simulink model "bicycle_20230612_Plots"  (R2022b)
settings: Solver=ode1  StartTime=0.0  StopTime=60  FixedStep=1e-4  RelTol=1e-3
model workspace (MAT data in the model file):
  Mu = [0.1; 0.1; 0; 0]
  x_init = [5; 0; 0]
libraries: simulink_extras x1
settings Model: Creator=giuli  LastModifiedBy=simob

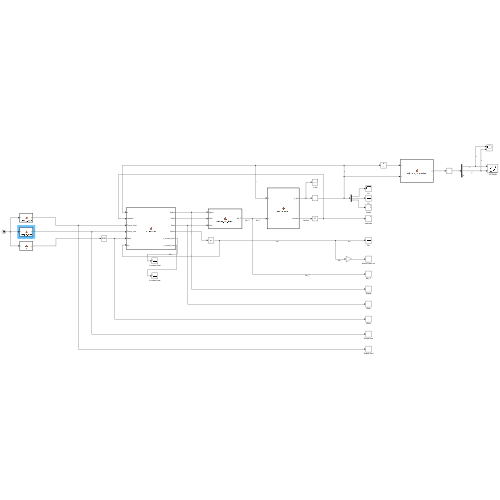
[thumbnail: Simulink's stored preview of the top-level diagram]
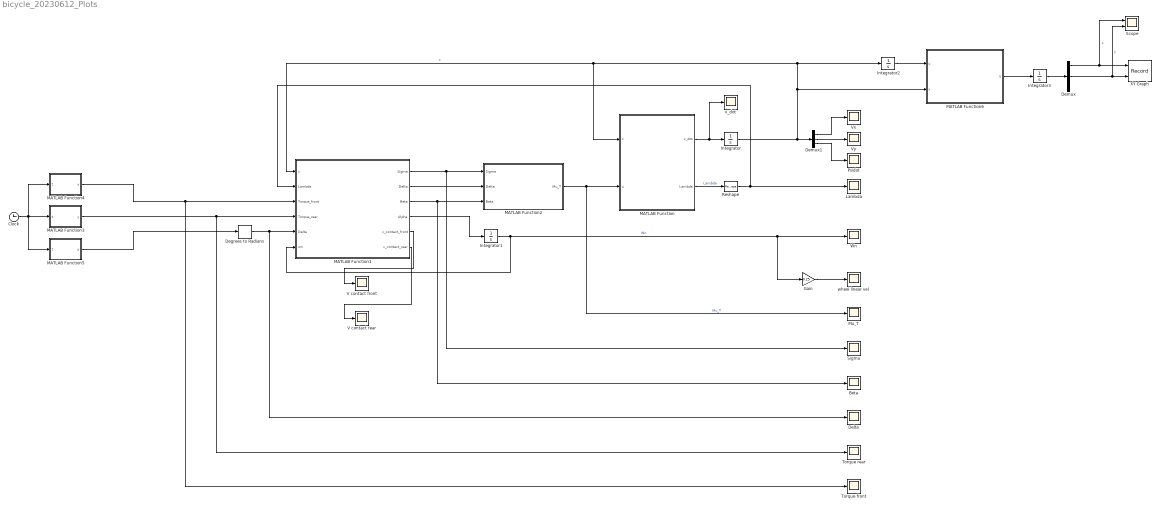
== system bicycle_20230612_Plots ==
  Beta : Scope
  Clock : Clock
  Degrees to Radians : simulink_extras/Transformations/Degrees to Radians
  Delta : Scope
  Demux : Demux  Outputs=3
  Demux1 : Demux  Outputs=3
  Gain : Gain  Gain=0.25
  Integrator : Integrator  InitialCondition=x_init
  Integrator1 : Integrator  InitialCondition=[x_init(1)/0.25; x_init(1)/0.25]
  Integrator2 : Integrator  InitialCondition=[0; 0; 0]
  Integrator3 : Integrator  InitialCondition=[0; 0; 0]
  Lambda : Scope
  MATLAB Function : MATLAB Function  TreatAsAtomicUnit=on
  MATLAB Function1 : MATLAB Function  TreatAsAtomicUnit=on
  MATLAB Function2 : MATLAB Function  TreatAsAtomicUnit=on
  MATLAB Function3 : MATLAB Function  TreatAsAtomicUnit=on
  MATLAB Function4 : MATLAB Function  TreatAsAtomicUnit=on
  MATLAB Function5 : MATLAB Function  TreatAsAtomicUnit=on
  MATLAB Function6 : MATLAB Function  TreatAsAtomicUnit=on
  Mu_T : Scope
  Psidot : Scope
  Reshape : Reshape  OutputDimensionality=Customize  OutputDimensions=[2,1]
  Scope : Scope  NumInputPorts=2
  Sigma : Scope
  Torque front : Scope
  Torque rear : Scope
  V contact front : Scope
  V contact rear : Scope
  Vx : Scope
  Vy : Scope
  Wn : Scope
  XY Graph : Record  FileSettingsInternal="{\"entries\":[{\"content\":{\"excelSettings\":{\"content\":{},\"type\":\"Streamout.ExcelSettings\"}},\"type\":\"Streamout.FileSettingStorage\",\"uuid\":\"d791e8b8-d0c3-44f8-9347-c5bd8d1bcd9f\"}],\"packageUris\":[\"http://schema.mathworks.com/mf0/streamout_blocks/R2020a\"],\"version\":\"1.0\"}"  Layout=[1 1]  SignalsInternal="{\"entries\":[{\"content\":{\"signals\":[{\"content\":{\"blockPath\":[\"bicycle_20230612/XY Graph\"],\"channel\":[],\"dimensions\":[1,1],\"domain\":\"bicycle_20230612/XY Graph\",\"lineColor\":\"#a2142f\",\"plots\":[1],\"port\":1,\"sid\":[\"\"],\"signalID\":16679,\"signalName\":\"x\"},\"type\":\"RecordBlkView.Signal\",\"uuid\":\"05d70a32-246a-412c-9d72-c4dce84ea26b\"},{\"content\":{\"blockPath\":[\"bicycle_20230612/XY Graph\"],\"channel\":[],\"dimensions\":[1,1],\"domain\":\"bicycle_20230612/XY Graph\",\"lineColor\":\"#139fff\",\"plots\":[1],\"port\":2,\"sid\":[\"\"],\"signalID\":16683,\"signalName\":\"y\"},\"type\":\"RecordBlkView.Signal\",\"uuid\":\"6831470b-3087-4cf1-ad87-be3c62b02656\"}]},\"type\":\"RecordBlkView.InputSignals\",\"uuid\":\"1d36ece6-da3a-41f1-b872-a8d311260c71\"}],\"packageUris\":[\"http://schema.mathworks.com/mf0/streamout_blocks/R2020a\"],\"version\":\"1.0\"}"  VisualizationBindings="{\"xyplotplugin\":{\"info\":[{\"series\":[{\"bindingParametersList\":[{\"parameter\":\"X-Axis\",\"signalID\":16679,\"signalName\":\"x\"},{\"parameter\":\"Y-Axis\",\"signalID\":16683,\"signalName\":\"y\"}],\"seriesID\":48522}],\"subplotID\":1}]}}"  CompatibilityTag=XY
  wheel linear vel : Scope
  x_dot : Scope
  wires:
  MATLAB Function/1(x_dot) -> Integrator/1, x_dot/1
  Integrator/1 -> Demux1/1, MATLAB Function6/2(x), Integrator2/1, MATLAB Function/1(x), MATLAB Function1/1(x)  "x"
  MATLAB Function/2(Lambda) -> Reshape/1  "Lambda"
  MATLAB Function2/1(Mu_T) -> Mu_T/1, MATLAB Function/2(u)  "Mu_T"
  MATLAB Function1/1(Sigma) -> MATLAB Function2/1(Sigma), Sigma/1
  MATLAB Function1/4(Alpha) -> Integrator1/1
  Integrator1/1 -> MATLAB Function1/6(wn), Gain/1, Wn/1  "Wn"
  MATLAB Function1/2(Delta) -> MATLAB Function2/2(Delta)
  MATLAB Function1/3(Beta) -> Beta/1, MATLAB Function2/3(Beta)
  Degrees to Radians/1 -> Delta/1, MATLAB Function1/5("Delta ")
  MATLAB Function5/1(y) -> Degrees to Radians/1
  Clock/1 -> MATLAB Function4/1(t), MATLAB Function5/1(t), MATLAB Function3/1(t)
  MATLAB Function3/1(y) -> Torque rear/1, MATLAB Function1/4(Torque_rear)
  Gain/1 -> wheel linear vel/1
  MATLAB Function4/1(y) -> MATLAB Function1/3(Torque_front), Torque front/1
  Integrator2/1 -> MATLAB Function6/1(u)
  MATLAB Function6/1(V) -> Integrator3/1
  Integrator3/1 -> Demux/1
  Demux/1 -> Scope/1, XY Graph/1  "x"
  Demux/2 -> Scope/2, XY Graph/2  "y"
  MATLAB Function1/5(v_contact_front) -> V contact front/1
  MATLAB Function1/6(v_contact_rear) -> V contact rear/1
  Reshape/1 -> MATLAB Function1/2(Lambda), Lambda/1
  Demux1/1 -> Vx/1
  Demux1/2 -> Vy/1
  Demux1/3 -> Psidot/1

== matlab function bicycle_20230612_Plots/MATLAB Function1 ==
  data: Sigma output; Delta output; Beta output; x input; Lambda input; Torque_front input; Torque_rear input; Delta input; Alpha output; wn input; v_contact_front output; v_contact_rear output
function [Sigma, Delta, Beta, Alpha, v_contact_front, v_contact_rear]  = tire_dynamics(x, Lambda, Torque_front, Torque_rear, Delta, wn)
%Alpha = [wn_front_dot, wn_rear_dot]

%%%
a = 1.421;
b = 1.029;

bfx = 8.22;
cfx = 1.65;
dfx = 1.688;
efx = -10;
r1fx = 13.476;
r2fx = 11.354;

brx = 8.22;
crx = 1.65;
drx = 1.688;
erx = -10;
r1rx = 13.476;
r2rx = 11.354;

cxbeta = 1.1231;
%%%

wheel_radius = 0.25; %m
wheel_mass = 15; %kg
wheel_Inertia = 0.5*wheel_mass*(wheel_radius^2); %cylinder inertia

torque_front = Torque_front;
torque_rear = Torque_rear;

wn_front = wn(1);
wn_rear = wn(2);

Vx = x(1);
Vy = x(2);
psi_dot = x(3);

%body frame
    psi_dot_skew = [0 -psi_dot 0; psi_dot 0 0; 0 0 0];
    v_contact_front = [Vx; Vy; 0] + psi_dot_skew*[a+b; 0; 0];
    v_contact_rear = [Vx; Vy; 0];

%sigma beta computation    
    beta_front = Delta-atan2(v_contact_front(2), v_contact_front(1));
    beta_rear = -atan2(v_contact_rear(2), v_contact_rear(1));
    Beta = [beta_front; beta_rear];

%wheel frame
    rotation_matrix = [cos(Delta) sin(Delta) 0; -sin(Delta) cos(Delta) 0; 0 0 1];
    v_contact_front = rotation_matrix*v_contact_front;
    % v_contact_rear is already fine
    sigma_front = (wheel_radius*wn_front - v_contact_front(1))/max(v_contact_front(1), wheel_radius*wn_front);
    sigma_rear = (wheel_radius*wn_rear - v_contact_rear(1))/max(v_contact_rear(1), wheel_radius*wn_rear);
    Sigma = [sigma_front; sigma_rear];

    fz_front = Lambda(1);
    fz_rear = Lambda(2);
    
    %angular velocities
    Mu_front = dfx*sin(cfx*atan(bfx*sigma_front-efx*(bfx*sigma_front-atan(bfx*sigma_front))))*cos(cxbeta*atan(beta_front*r1fx/(1+(r2fx*sigma_front)^2)));%in wheel frame
    Mu_rear = drx*sin(crx*atan(brx*sigma_rear-erx*(brx*sigma_rear-atan(brx*sigma_rear))))*cos(cxbeta*atan(beta_rear*r1rx/(1+(r2rx*sigma_rear)^2)));%in wheel frame
    Fx_front = -fz_front*Mu_front; %-
    Fx_rear = -fz_rear*Mu_rear; %-

    alpha_front = (torque_front - wheel_radius*Fx_front)/wheel_Inertia;
    alpha_rear = (torque_rear - wheel_radius*Fx_rear)/wheel_Inertia;
    Alpha = [alpha_front; alpha_rear];

    Mu = [Mu_front; Mu_rear];

== matlab function bicycle_20230612_Plots/MATLAB Function ==
  data: x input; u input; x_dot output; Lambda output
function [x_dot, Lambda] = car_dynamics(x,u)
m = 1480;
a = 1.421;
b = 1.029;
h = 0.42;
g = 9.81;
Izz = 1950;
Ixz = -50;

Vx = x(1);
Vy = x(2);
Psi_dot = x(3);

MuFx = u(1);
MuRx = u(2);
MuFy = u(3);
MuRy = u(4);

M = [m 0 0 MuFx MuRx;
    0 m m*b MuFy MuRy;
    0 m*b (Izz+m*(b^2)) (a+b)*MuFy 0;
    0 0 0 -1 -1;
    -m*h 0 0 a+b 0];

K = [-m*b*(Psi_dot^2)-m*Vy*Psi_dot;
    m*Vx*Psi_dot;
    m*b*Vx*Psi_dot;
    -m*g;
    (Ixz+m*h*b)*(Psi_dot^2)+m*h*Vy*Psi_dot+m*g*b];

out = -inv(M)*K;

x_dot = out(1:3);
Lambda = out(4:5);

== matlab function bicycle_20230612_Plots/MATLAB Function2 ==
  data: Sigma input; Mu_T output; Delta input; Beta input
function Mu_T = Pacejka_tire_model(Sigma, Delta, Beta)
%%%
bfx = 8.22;
cfx = 1.65;
dfx = 1.688;
efx = -10;
r1fx = 13.476;
r2fx = 11.354;

brx = 8.22;
crx = 1.65;
drx = 1.688;
erx = -10;
r1rx = 13.476;
r2rx = 11.354;

bfy = 12.848;
cfy = 1.79;
dfy = 1.688;
efy = -1.206;
r1fy = 7.7856;
r2fy = 8.1697;

bry = 8.822;
cry = 1.79;
dry = 1.688;
ery = -2.02;
r1ry = 7.7856;
r2ry = 8.1697;

cxbeta = 1.1231;
cysigma = 1.0533;
%%%

%%%
beta_front = Beta(1);
beta_rear = Beta(2);

sigma_front = Sigma(1);
sigma_rear = Sigma(2);
%%%

MuFx = F0_fnc(sigma_front, bfx, cfx, dfx, efx) * Gx_fnc(sigma_front, beta_front, cxbeta, r1fx, r2fx);
MuRx = F0_fnc(sigma_rear, brx, crx, drx, erx) * Gx_fnc(sigma_rear, beta_rear, cxbeta, r1rx, r2rx);
MuFy = F0_fnc(beta_front, bfy, cfy, dfy, efy) * Gy_fnc(sigma_front, beta_front, cysigma, r1fy, r2fy);
MuRy = F0_fnc(beta_rear, bry, cry, dry, ery) * Gy_fnc(sigma_rear, beta_rear, cysigma, r1ry, r2ry);

MuFx_T = MuFx*cos(Delta) - MuFy*sin(Delta);
MuRx_T = MuRx;
MuFy_T = MuFx*sin(Delta) + MuFy*cos(Delta);
MuRy_T = MuRy;

Mu_T = [MuFx_T MuRx_T MuFy_T MuRy_T];
end

function Gy = Gy_fnc(Sigma, Beta, cysigma, r1, r2) 
    Gy = cos(cysigma*atan(Sigma*r1/(1+(r2*Beta)^2)));
end

function F0 = F0_fnc(x, b, c, d, e)
    F0 = d*sin(c*atan(b*x-e*(b*x-atan(b*x))));
end

function Gx = Gx_fnc(Sigma, Beta, cxbeta, r1, r2) 
    Gx = cos(cxbeta*atan(Beta*r1/(1+(r2*Sigma)^2)));
end

== matlab function bicycle_20230612_Plots/MATLAB Function3 ==
  data: t input; y output
function y = Torque_rear(t)

y = 300;
end

== matlab function bicycle_20230612_Plots/MATLAB Function4 ==
  data: t input; y output
function y = Torque_front(t)
% 
% if t > 10
%      y = -100;
% else
%      y = 0;
% end

% y = 500*exp((t-5)^2/100);

y = 300;

end

== matlab function bicycle_20230612_Plots/MATLAB Function5 ==
  data: t input; y output
function y = Delta(t)

if t > 10
     y = 3;
else
     y = 0.3*t;
end
% y = 0.1*t;
% end

== matlab function bicycle_20230612_Plots/MATLAB Function6 ==
  data: u input; x input; V output
function V = trajectory_computation(u,x)
psi = u(3);
Vx = x(1);
Vy = x(2);

%body frame
Vx_vect = [Vx; 0; 0];
Vy_vect = [0; Vy; 0];

%global frame
rotation_matrix = [cos(psi) sin(psi) 0; sin(psi) -cos(psi) 0; 0 0 1];
Vx_vect = rotation_matrix*Vx_vect;
Vy_vect = rotation_matrix*Vy_vect;
V = Vx_vect + Vy_vect;
